simulink model "PV_Model_4thstring_shuffle_mppt"  (R2018a)
settings: Solver=FixedStepDiscrete  StartTime=0.0  StopTime=2  RelTol=1e-3
libraries: powerlib x37, re_lib x6
settings Model: Creator=burge  LastModifiedBy=burge
settings DataIOCC: SaveState=on

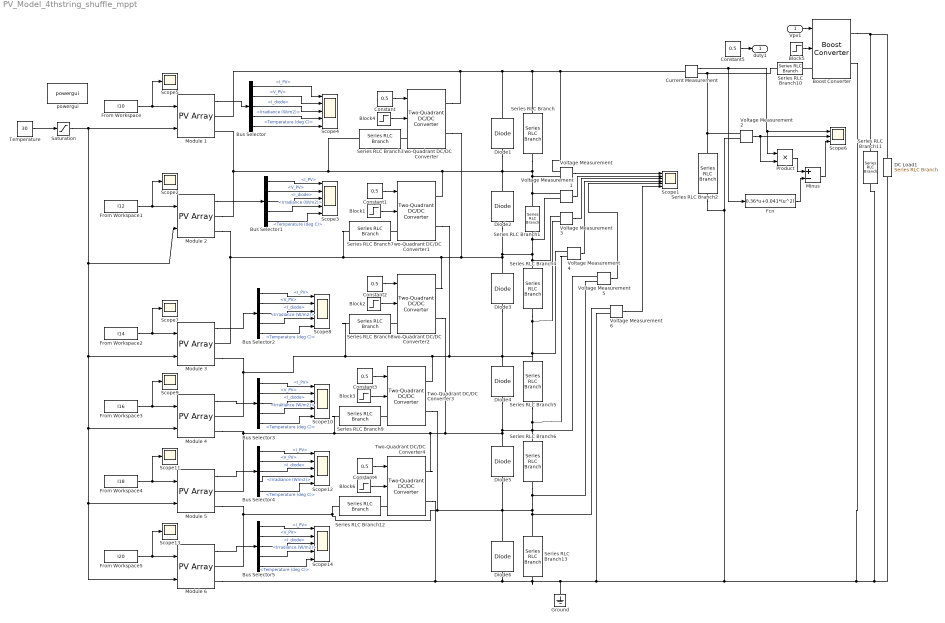
== system PV_Model_4thstring_shuffle_mppt ==
  Vpv1 : Inport  OutDataTypeStr=double  PortDimensions=1  SampleTime=[0.0001,0]
  Block{1..6} (6 alike) : Step  Time=0  Before=1  After=0  SampleTime=5e-5
  Boost Converter : powerlib/Power Electronics/Boost Converter  ModelType=Average model (D-controlled)  Ron=1e-3  Rs=1e6  Cs=inf  Vforward=[0,0]  Ron_Diode=1e-3  Rs_Diode=1e6  Cs_Diode=inf  Vf_Diode=1e-3  Rs_CurrentSource=inf
      settings: SourceProductName=Simscape Power Systems  SourceProductBaseCode=PS
  Bus Selector{,1..5} (6 alike) : BusSelector  OutputSignals=I_PV,V_PV,I_diode,Irradiance (W/m2),Temperature (deg C)
  Constant{,1..5} (6 alike) : Constant  Value=0.5
  Current Measurement : powerlib/Measurements/Current Measurement  PhasorSimulation=off  OutputType=Complex  PSBequivalent=0
  DC Load1 : powerlib/Elements/Series RLC Branch  LConnTagsString=__new0  RConnTagsString=__new0  BranchType=R  Resistance=13  Inductance=1e-3  SetiL0=off  InitialCurrent=0  Capacitance=1e-6  Setx0=off  InitialVoltage=0  Measurements=None
  Diode{1..6} (6 alike) : powerlib/Power Electronics/Diode  Ron=0.05  Lon=0  Vf=0.7  IC=0  UseSnubber=0  Rs=500  Cs=250e-9  Measurements=off
  Fcn : Fcn  Expr=0.36*u+0.041*(u^2)
  From Workspace : FromWorkspace  VariableName=I10  OutDataTypeStr=double  SampleTime=0  OutputAfterFinalValue=Holding final value
  From Workspace1 : FromWorkspace  VariableName=I12  OutDataTypeStr=double  SampleTime=0  OutputAfterFinalValue=Holding final value
  From Workspace2 : FromWorkspace  VariableName=I14  OutDataTypeStr=double  SampleTime=0  OutputAfterFinalValue=Holding final value
  From Workspace3 : FromWorkspace  VariableName=I16  OutDataTypeStr=double  SampleTime=0  OutputAfterFinalValue=Holding final value
  From Workspace4 : FromWorkspace  VariableName=I18  OutDataTypeStr=double  SampleTime=0  OutputAfterFinalValue=Holding final value
  From Workspace5 : FromWorkspace  VariableName=I20  OutDataTypeStr=double  SampleTime=0  OutputAfterFinalValue=Holding final value
  Ground : powerlib/Elements/Ground  LConnTagsString=a
  Minus : Sum  Inputs=+-
  Module {1..6} (6 alike) : re_lib/Solar/PV Array  Npar=1  Nser=12  PlotType=array @ 1000 W/m2 & specified temperatures  S_vec="[ 1000  500  100 ]"  Temp_C_vec="[ 45 25  ]"  ModuleName=User-defined  PlotWhenSelected=off  Pm=3.8912  Ncell=1  Voc=0.727  Isc=6.45  Vm=0.64  Im=6.08  beta_Voc_pc=-0.2393  alpha_Isc_pc=0.045  beta_Voc=-0.0017397  alpha_Isc=0.0029025  IL=6.4807  I0=1.3352e-12  nI=0.96977  Rsh=3.547  Rs=0.00078547  BAL=on  Tc=1e-6  Tfilter=5e-5
  Product : Product
  Saturation : Saturate  UpperLimit=55  LowerLimit=5
  Scope1 : Scope  NumInputPorts=6
  Scope{3..4,8,10,12,14} (6 alike) : Scope  NumInputPorts=5
  Scope{2,5,7,9,11,13} (6 alike) : Scope
  Scope6 : Scope  NumInputPorts=3
  Series RLC Branch{,1,4..6,11,13} (7 alike) : powerlib/Elements/Series RLC Branch  LConnTagsString=__new0  RConnTagsString=__new0  BranchType=C  Resistance=1  Inductance=1e-3  SetiL0=off  InitialCurrent=0  Capacitance=100e-6  Setx0=off  InitialVoltage=0  Measurements=None
  Series RLC Branch10 : powerlib/Elements/Series RLC Branch  LConnTagsString=__new0  RConnTagsString=__new0  BranchType=L  Resistance=1  Inductance=1e-4  SetiL0=off  InitialCurrent=0  Capacitance=1e-6  Setx0=off  InitialVoltage=0  Measurements=None
  Series RLC Branch{3,7..9,12} (5 alike) : powerlib/Elements/Series RLC Branch  LConnTagsString=__new0  RConnTagsString=__new0  BranchType=RL  Resistance=0.01  Inductance=1e-4  SetiL0=off  InitialCurrent=0  Capacitance=1e-6  Setx0=off  InitialVoltage=0  Measurements=None
  Series RLC Branch2 : powerlib/Elements/Series RLC Branch  LConnTagsString=__new0  RConnTagsString=__new0  BranchType=C  Resistance=1  Inductance=1e-3  SetiL0=off  InitialCurrent=0  Capacitance=10000e-6  Setx0=off  InitialVoltage=0  Measurements=None
  Temperature : Constant  Value=30
  Two-Quadrant DC/DC Converter{,1..4} (5 alike) : powerlib/Power Electronics/Two-Quadrant DC//DC Converter  ModelType=Average model (D-controlled)  Ron=1e-3  Rs=1e6  Cs=inf  Vforward=[0,0]  Ron_Diode=1e-3  Rs_Diode=1e6  Cs_Diode=inf  Vf_Diode=1e-3  Rs_CurrentSource=inf
      settings: SourceProductName=Simscape Power Systems  SourceProductBaseCode=PS
  Voltage Measurement{,1..6} (7 alike) : powerlib/Measurements/Voltage Measurement  PhasorSimulation=off  OutputType=Complex  PSBequivalent=0
  powergui : powerlib/powergui  Priority=1  SimulationMode=Discrete  SampleTime=5e-6  frequency=60  Iterations=50  frequencyindice=0  Pbase=100e6  ErrMax=1e-4  UnitsV=kV  UnitsW=MW  buscounter=0  FunctionMessages=off  echomessages=off  EnableUseOfTLC=off  CurrentSourceSwitches=off  DisableSnubberDevices=off  DisableRonSwitches=off  DisableVfSwitches=off  DisplayEquations=off  SolverType=Tustin/Backward Euler (TBE)  Interpol=off  ExternalGateDelay=off  methode=off  Ts=100  x0status=blocks  SPID=off  SwTol=0  HookPort=off  RestoreLinks=warning  ResistiveCurrentMeasurement=off  Frange=[0:2:500]  Ylog=off  Xlog=on  ShowGrid=off  save=off  variable=ZData  structure=0  ZoomFFT=off  StartTime=0.0  cycles=1  DisplayStyle=1  fundamental=60  FreqAxis=off  MaxFrequency=1000  frequencyindicesteady=1  RmsSteady=1  display=off
  duty1 : Outport  OutDataTypeStr=double  PortDimensions=1  SampleTime=[0.0001,0]
  wires:
  Module 1/1 -> Bus Selector/1
  Bus Selector/1 -> Scope4/1  "<I_PV>"
  From Workspace/1 -> Scope5/1, Module 1/1
  Temperature/1 -> Saturation/1
  Bus Selector/2 -> Scope4/2  "<V_PV>"
  Bus Selector/3 -> Scope4/3  "<I_diode>"
  Bus Selector/4 -> Scope4/4  "<Irradiance (W/m2)>"
  Bus Selector/5 -> Scope4/5  "<Temperature (deg C)>"
  Voltage Measurement/1 -> Scope1/1
  Saturation/1 -> Module 6/2, Module 5/2, Module 4/2, Module 3/2, Module 2/2, Module 1/2
  From Workspace1/1 -> Scope2/1, Module 2/1
  Bus Selector1/4 -> Scope3/4  "<Irradiance (W/m2)>"
  Bus Selector1/5 -> Scope3/5  "<Temperature (deg C)>"
  Bus Selector1/2 -> Scope3/2  "<V_PV>"
  Bus Selector1/3 -> Scope3/3  "<I_diode>"
  Module 2/1 -> Bus Selector1/1
  Bus Selector1/1 -> Scope3/1  "<I_PV>"
  Voltage Measurement1/1 -> Scope1/2
  Voltage Measurement2/1 -> Product/2, Scope6/2
  Current Measurement/1 -> Fcn/1, Product/1, Scope6/1
  Constant/1 -> Two-Quadrant DC/DC Converter/1
  Block4/1 -> Two-Quadrant DC/DC Converter/2
  From Workspace2/1 -> Scope7/1, Module 3/1
  Bus Selector2/1 -> Scope8/1  "<I_PV>"
  Bus Selector2/5 -> Scope8/5  "<Temperature (deg C)>"
  Bus Selector2/4 -> Scope8/4  "<Irradiance (W/m2)>"
  Bus Selector2/3 -> Scope8/3  "<I_diode>"
  Bus Selector2/2 -> Scope8/2  "<V_PV>"
  Module 3/1 -> Bus Selector2/1
  Voltage Measurement3/1 -> Scope1/3
  From Workspace3/1 -> Scope9/1, Module 4/1
  Bus Selector3/2 -> Scope10/2  "<V_PV>"
  Bus Selector3/4 -> Scope10/4  "<Irradiance (W/m2)>"
  Bus Selector3/5 -> Scope10/5  "<Temperature (deg C)>"
  Bus Selector3/1 -> Scope10/1  "<I_PV>"
  Bus Selector3/3 -> Scope10/3  "<I_diode>"
  Module 4/1 -> Bus Selector3/1
  Voltage Measurement4/1 -> Scope1/4
  From Workspace4/1 -> Scope11/1, Module 5/1
  Bus Selector4/3 -> Scope12/3  "<I_diode>"
  Bus Selector4/4 -> Scope12/4  "<Irradiance (W/m2)>"
  Bus Selector4/5 -> Scope12/5  "<Temperature (deg C)>"
  Bus Selector4/2 -> Scope12/2  "<V_PV>"
  Module 5/1 -> Bus Selector4/1
  Bus Selector4/1 -> Scope12/1  "<I_PV>"
  Voltage Measurement5/1 -> Scope1/5
  Block1/1 -> Two-Quadrant DC/DC Converter1/2
  Constant1/1 -> Two-Quadrant DC/DC Converter1/1
  Block2/1 -> Two-Quadrant DC/DC Converter2/2
  Constant2/1 -> Two-Quadrant DC/DC Converter2/1
  Block3/1 -> Two-Quadrant DC/DC Converter3/2
  Constant3/1 -> Two-Quadrant DC/DC Converter3/1
  Block5/1 -> Boost Converter/2
  Vpv1/1 -> Boost Converter/1
  From Workspace5/1 -> Scope13/1, Module 6/1
  Bus Selector5/3 -> Scope14/3  "<I_diode>"
  Bus Selector5/1 -> Scope14/1  "<I_PV>"
  Bus Selector5/2 -> Scope14/2  "<V_PV>"
  Bus Selector5/5 -> Scope14/5  "<Temperature (deg C)>"
  Bus Selector5/4 -> Scope14/4  "<Irradiance (W/m2)>"
  Module 6/1 -> Bus Selector5/1
  Block6/1 -> Two-Quadrant DC/DC Converter4/2
  Constant4/1 -> Two-Quadrant DC/DC Converter4/1
  Voltage Measurement6/1 -> Scope1/6
  Constant5/1 -> duty1/1
  Fcn/1 -> Minus/2
  Product/1 -> Minus/1
  Minus/1 -> Scope6/3
  connections:
  Module 2/RConn1 -- Series RLC Branch3/LConn1 -- Two-Quadrant DC/DC Converter1/RConn1 -- Series RLC Branch1/LConn1 -- Voltage Measurement1/LConn1 -- Voltage Measurement/LConn2 -- Series RLC Branch/RConn1 -- Diode2/RConn1 -- Diode1/LConn1 -- Module 1/RConn2
  Voltage Measurement2/LConn1 -- Series RLC Branch10/LConn1 -- Current Measurement/RConn1 -- Series RLC Branch2/LConn1
  Series RLC Branch3/RConn1 -- Two-Quadrant DC/DC Converter/LConn1
  Module 2/RConn2 -- Series RLC Branch7/LConn1 -- Two-Quadrant DC/DC Converter2/RConn1 -- Two-Quadrant DC/DC Converter/RConn2 -- Voltage Measurement3/LConn1 -- Series RLC Branch4/LConn1 -- Voltage Measurement1/LConn2 -- Series RLC Branch1/RConn1 -- Diode2/LConn1 -- Diode3/RConn1 -- Module 3/RConn1
  Series RLC Branch4/RConn1 -- Voltage Measurement3/LConn2 -- Voltage Measurement4/LConn1 -- Diode3/LConn1 -- Two-Quadrant DC/DC Converter1/RConn2 -- Two-Quadrant DC/DC Converter3/RConn1 -- Series RLC Branch8/LConn1 -- Module 4/RConn1 -- Module 3/RConn2 -- Diode4/RConn1 -- Series RLC Branch5/LConn1
  Series RLC Branch5/RConn1 -- Voltage Measurement4/LConn2 -- Series RLC Branch9/LConn1 -- Module 5/RConn1 -- Module 4/RConn2 -- Two-Quadrant DC/DC Converter4/RConn1 -- Two-Quadrant DC/DC Converter2/RConn2 -- Diode5/RConn1 -- Diode4/LConn1 -- Voltage Measurement5/LConn1 -- Series RLC Branch6/LConn1
  Series RLC Branch/LConn1 -- Current Measurement/LConn1 -- Voltage Measurement/LConn1 -- Two-Quadrant DC/DC Converter/RConn1 -- Module 1/RConn1 -- Diode1/RConn1
  Series RLC Branch7/RConn1 -- Two-Quadrant DC/DC Converter1/LConn1
  Series RLC Branch8/RConn1 -- Two-Quadrant DC/DC Converter2/LConn1
  Series RLC Branch9/RConn1 -- Two-Quadrant DC/DC Converter3/LConn1
  Boost Converter/LConn1 -- Series RLC Branch10/RConn1
  Boost Converter/RConn1 -- DC Load1/LConn1 -- Series RLC Branch11/LConn1
  Diode5/LConn1 -- Two-Quadrant DC/DC Converter3/RConn2 -- Series RLC Branch12/LConn1 -- Module 5/RConn2 -- Module 6/RConn1 -- Diode6/RConn1 -- Voltage Measurement6/LConn1 -- Series RLC Branch13/LConn1 -- Voltage Measurement5/LConn2 -- Series RLC Branch6/RConn1
  Series RLC Branch12/RConn1 -- Two-Quadrant DC/DC Converter4/LConn1
  Boost Converter/RConn2 -- Series RLC Branch11/RConn1 -- DC Load1/RConn1 -- Ground/LConn1 -- Series RLC Branch13/RConn1 -- Diode6/LConn1 -- Two-Quadrant DC/DC Converter4/RConn2 -- Module 6/RConn2 -- Voltage Measurement6/LConn2 -- Series RLC Branch2/RConn1 -- Voltage Measurement2/LConn2
